simulink model "collaborative_robot2"  (R2021a)
settings: Solver=VariableStepAuto  StartTime=0.0  StopTime=inf  RelTol=1e-3
libraries: vrlib x1, simulink x1
settings Model: Creator=kbhar  LastModifiedBy=kbhar

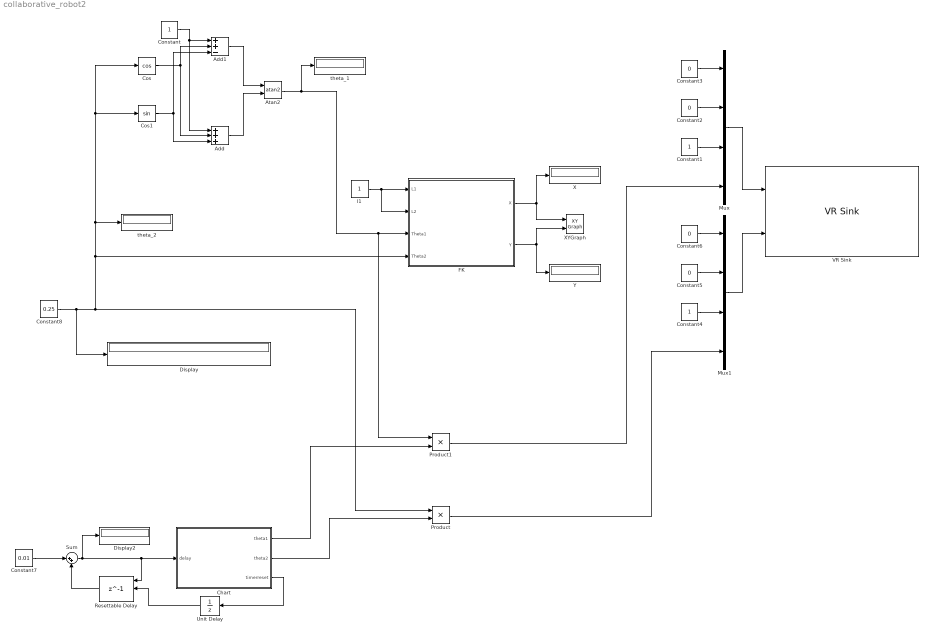
== system collaborative_robot2 ==
  Add : Sum  Inputs=+++
  Add1 : Sum  Inputs=++-
  Atan2 : Trigonometry  Operator=atan2
  Chart : Stateflow chart  TreatAsAtomicUnit=on
  Constant : Constant
  Constant1 : Constant
  Constant{2..3,5..6} (4 alike) : Constant  Value=0
  Constant4 : Constant
  Constant7 : Constant  Value=0.01
  Constant8 : Constant  Value=0.25
  Cos : Trigonometry  Operator=cos
  Cos1 : Trigonometry
  Display : Display
  Display2 : Display
  FK : Subsystem
  Mux : Mux
  Mux1 : Mux
  Product : Product
  Product1 : Product
  Resettable Delay : Delay  DelayLength=1  InitialConditionSource=Input port  ExternalReset=Rising
      settings: InputPortMap=u0,r5,p4
  Sum : Sum  Inputs=|++
  Unit Delay : UnitDelay  SampleTime=-1  HasFrameUpgradeWarning=on
  VR Sink : vrlib/VR Sink  InstantiateOnLoad=on  SampleTime=0.1  ViewEnable=on  RemoteChange=off  RemoteView=off  FieldsWritten=shoulder_joint.rotation.4.1.1.double#elbow_joint.rotation.4.1.1.double  WorldFileName=C:\Bharat\College\Projects\Arm Control\Files\test_two_joint_arm.wrl  AutoView=off  VideoDimensions=[]  AllowVariableSize=off
  X : Display
  XYGraph : simulink/Sinks/XY Graph  xmin=-1  xmax=2  ymin=-1  ymax=2  st=-1
  Y : Display
  l1 : Constant
  theta_1 : Display
  theta_2 : Display
  wires:
  Constant/1 -> Add1/1, Add/1
  Cos/1 -> Add/2, Add1/2
  Cos1/1 -> Add/3, Add1/3
  Add1/1 -> Atan2/1
  Add/1 -> Atan2/2
  Constant4/1 -> Mux1/3
  Constant5/1 -> Mux1/2
  Atan2/1 -> FK/3(Theta1), Product1/1, theta_1/1
  Constant3/1 -> Mux/1
  Constant1/1 -> Mux/3
  Mux/1 -> VR Sink/1
  Mux1/1 -> VR Sink/2
  Constant2/1 -> Mux/2
  Constant6/1 -> Mux1/1
  Constant8/1 -> Display/1, Cos/1, Cos1/1, theta_2/1, FK/4(Theta2), Product/1
  FK/1(X) -> XYGraph/1, X/1
  l1/1 -> FK/2(L2), FK/1(L1)
  FK/2(Y) -> XYGraph/2, Y/1
  Unit Delay/1 -> Resettable Delay/2
  Resettable Delay/1 -> Sum/2
  Constant7/1 -> Sum/1
  Sum/1 -> Display2/1, Chart/1(delay), Resettable Delay/1
  Chart/3(timerreset) -> Unit Delay/1
  Chart/2(theta2) -> Product/2
  Chart/1(theta1) -> Product1/2
  Product1/1 -> Mux/4
  Product/1 -> Mux1/4

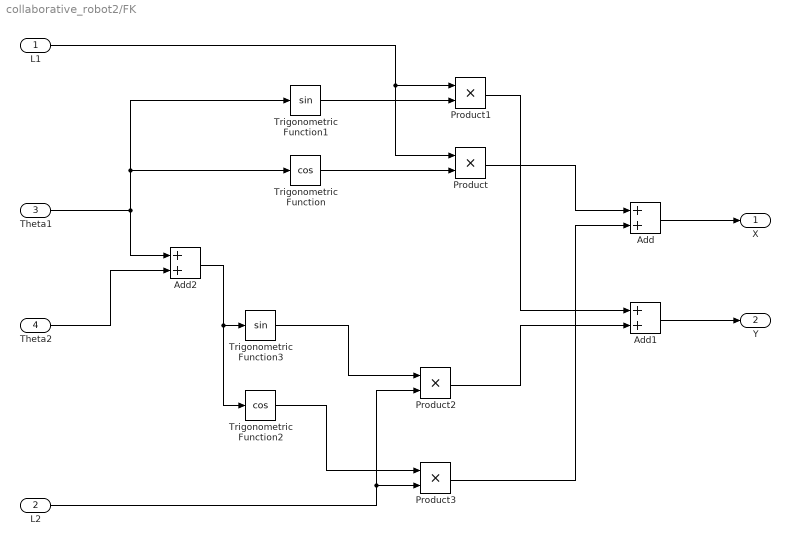
== system collaborative_robot2/FK ==
  L1 : Inport
  L2 : Inport  Port=2
  Theta1 : Inport  Port=3
  Theta2 : Inport  Port=4
  Add : Sum
  Add1 : Sum
  Add2 : Sum
  Product{,1..3} (4 alike) : Product
  Trigonometric Function : Trigonometry  Operator=cos
  Trigonometric Function1 : Trigonometry
  Trigonometric Function2 : Trigonometry  Operator=cos
  Trigonometric Function3 : Trigonometry
  X : Outport
  Y : Outport  Port=2
  wires:
  Trigonometric Function1/1 -> Product1/2
  Trigonometric Function2/1 -> Product3/1
  Product1/1 -> Add1/1
  Add2/1 -> Trigonometric Function3/1, Trigonometric Function2/1
  L1/1 -> Product/1, Product1/1
  Trigonometric Function3/1 -> Product2/1
  Theta1/1 -> Trigonometric Function1/1, Trigonometric Function/1, Add2/1
  Trigonometric Function/1 -> Product/2
  Product/1 -> Add/1
  L2/1 -> Product2/2, Product3/2
  Product2/1 -> Add1/2
  Product3/1 -> Add/2
  Add/1 -> X/1
  Theta2/1 -> Add2/2
  Add1/1 -> Y/1

== stateflow chart collaborative_robot2/Chart ==
  state startstate
    theta1 = 0; theta2 = 0; timerreset = 0;
  state usercontrolstate
    theta1 = 0; theta2 = 1; timerreset = 0;
  state resetstate
    theta1 = 0; theta2 = 0; timerreset = 1;
  state robotcontrolstate
    theta1 = 1; theta2 = 1; timerreset = 0;
  (default) -> startstate
  startstate -> usercontrolstate
  resetstate -> usercontrolstate
  usercontrolstate -> robotcontrolstate : [delay > 25]
  robotcontrolstate -> resetstate : [delay > 75]
  data: delay input; theta1 output; theta2 output; timerreset output
